simulink model "mympc15a"  (R2015a)
settings: Solver=ode45  SolverMode=SingleTasking  StartTime=0.0  StopTime=10.0  RelTol=1e-3
settings Model: CovMetricSettings=dwe  CovHtmlReporting=off  covSaveCumulativeToWorkspaceVar=off  CovSaveSingleToWorkspaceVar=off  CovExternalEMLEnable=on  Creator=mati  LastModifiedBy=mati
settings DataIOCC: LimitDataPoints=off  SaveFormat=Dataset  ReturnWorkspaceOutputs=on
settings DebuggingCC: UnconnectedInputMsg=none  UnconnectedOutputMsg=none  UnconnectedLineMsg=none  SFUnexpectedBacktrackingDiag=error  SFNoUnconditionalDefaultTransitionDiag=error
settings HardwareCC: ProdBitPerPointer=64  ProdLargestAtomicFloat=Float  ProdIntDivRoundTo=Zero  ProdEndianess=LittleEndian  ProdHWDeviceType=Specified
settings ModelReferenceCC: PropagateSignalLabelsOutOfModel=on
settings SFSimCC: SimUseLocalCustomCode=on
settings RTWCC: RTWUseLocalCustomCode=on
settings GRTTargetCC: TargetLangStandard=C99 (ISO)

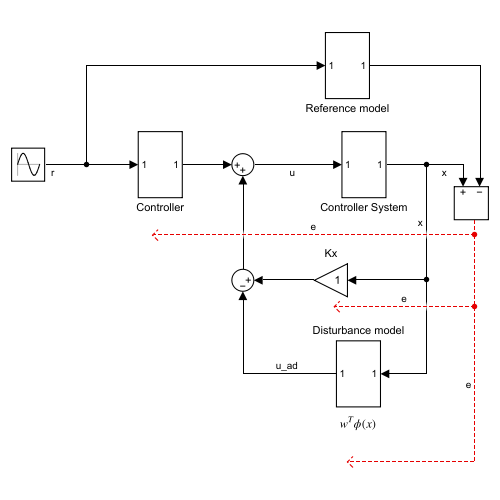
[thumbnail: Simulink's stored preview of the top-level diagram]
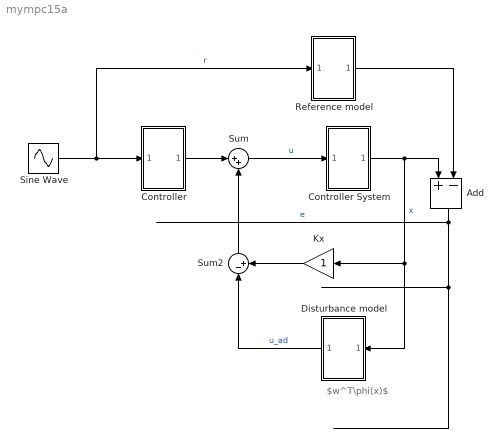
== system mympc15a ==
  note: $w^T\phi(x)$
  Add : Sum  Inputs=+-
  Controller : Subsystem
  Controller System : Subsystem
  Disturbance model : Subsystem
  Kx : Gain
  Reference model : Subsystem
  Sine Wave : Sin  SampleTime=0
  Sum : Sum  Inputs=|++
  Sum2 : Sum  Inputs=|-+
  wires:
  Sine Wave/1 -> Reference model/1(In1), Controller/1(In1)  "r"
  Controller/1(Out1) -> Sum/1
  Sum2/1 -> Sum/2
  Sum/1 -> Controller System/1(In1)  "u"
  Controller System/1(Out1) -> Disturbance model/1(In1), Kx/1, Add/1  "x"
  Reference model/1(Out1) -> Add/2
  Kx/1 -> Sum2/2
  Disturbance model/1(Out1) -> Sum2/1  "u_ad"
  Add/1 -> ?  "e"

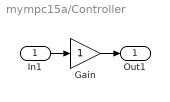
== system mympc15a/Controller ==
  In1 : Inport
  Gain : Gain
  Out1 : Outport
  wires:
  In1/1 -> Gain/1
  Gain/1 -> Out1/1

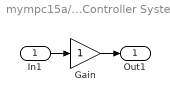
== system mympc15a/Controller System ==
  In1 : Inport
  Gain : Gain
  Out1 : Outport
  wires:
  In1/1 -> Gain/1
  Gain/1 -> Out1/1

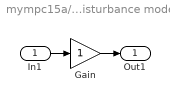
== system mympc15a/Disturbance model ==
  In1 : Inport
  Gain : Gain
  Out1 : Outport
  wires:
  In1/1 -> Gain/1
  Gain/1 -> Out1/1

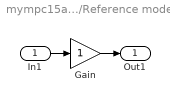
== system mympc15a/Reference model ==
  In1 : Inport
  Gain : Gain
  Out1 : Outport
  wires:
  In1/1 -> Gain/1
  Gain/1 -> Out1/1
